simulink model "V2X_Core_SRI_coding_rate_symbol"  (R2023b)
settings: Solver=ode23tb  StartTime=0.0  StopTime=50  MaxStep=1e-2  RelTol=1e-3  AbsTol=1e-3
StopFcn:
  | run('saving.m')
values from neighbouring files (symbols this model uses):
  b = 1.6    [a2024_v2x_matlab_6veh.m]
  m = 2000    [a2024_v2x_matlab_6veh.m]
  mEgo = 1500    [a2024_v2x_matlab_6veh.m]
  Mode = 1    [a2024_v2x_matlab_6veh.m]    (also in v2x_matlab.m; v2x_matlabV2.m; v2x_matlab_6veh.m; v2x_matlab_R.m)
  RefSpeed = 90/3.6    (= 25)    [v2x_matlabV2.m]    (also in v2x_matlab_R.m)
  RelDistThreshold = 300    [v2x_matlabV2.m]    (also in v2x_matlab_R.m)
  s = RandStream("dsfmt19937","Seed",15)    [v2x_matlab.m]
  sampleTime = 0.1    [a2024_v2x_matlab_6veh.m]    (also in v2x_matlab.m; v2x_matlabV2.m; v2x_matlab_6veh.m; v2x_matlab_R.m)
  waypoints = [egoWP(:,2) egoWP(:,1), zeroforwp]    [a2024_v2x_matlab_6veh.m]    (also in misc.m = data.data.ActorSpecifications(1,1).Waypoints(:,[1,2]); v2x_matlab.m = data.data.ActorSpecifications(1,1).Waypoints(:,[1,2]); v2x_matlabV2.m = [5 -1.6 0; v2x_matlab_R.m = [5 -1.6 0)
  ZeroActors = struct(     'ActorID',0,     'Position', [1000 1000 1000],      'Velocity', [0 0 0],      'Roll', 0,      'Pitch', 0,      'Yaw', 0,      'AngularVelocity', [0 0 0])    [v2x_matlabV2.m]    (also in v2x_matlab_R.m)
undefined symbols (not defined in the file or in its folder): Battery, Brakes, Control, DiscIntNeverNeededParam, doppler, Drivetrain, ElectricMotor, Env, FB_flag, Init, SNR_value_list, Vehicle, Wheels
libraries: simulink x45, commofdm x29, commdigbbndam3 x15, commchan3 x14, simulink_extras x13, commcnvcod2 x12, commdigbbndpm3 x11, commblkintrlv2 x10, dspmathops x6, sharedtransform x6, autolibutils x6, autolibsharedcoupling x4
(part 8 of 8)

== matlab function V2X_Core_SRI_coding_rate_symbol/Calculate PDR/PDR V5/MATLAB Function ==
  settings: updateMethod=DISCRETE  sampleTime=sampleTime
  data: Tx input; PDR output; Rx input; Rx_out output; Msg_out output
function [PDR, Rx_out, Msg_out] = PDR(Tx, Rx)
    persistent N S prev_Rx
    if isempty(N) || isempty(S)
        N = 0;
        S = 0;
        prev_Rx = zeros(13,1);
    end
    if isequal(Tx, Rx) % Check if the entire vectors are the same
        N = N + 1;      % Increment the correct packet count
        prev_Rx = Rx;
        Rx_out = Rx;
        Msg_out = 1;
    else
        Rx_out = prev_Rx;
        Msg_out = 0;
    end
    S = S + 1;          % Increment the total count
    R = (N/S)*100;       % Calculate the packet delivery rate [%]
    PDR = [R; N; S];
end

== matlab function V2X_Core_SRI_coding_rate_symbol/Calculate PDR/PDR V5/MATLAB Function1 ==
  settings: sampleTime=sampleTime
  data: Vehicle_ID input; u input; y output double
function y = fcn(Vehicle_ID, u)

if isempty(u(:,Vehicle_ID)) 
    y = zeros(1,15);
else
    y = double(u(:,Vehicle_ID));
end

end

== matlab function V2X_Core_SRI_coding_rate_symbol/Calculate PDR/PDR V5/MATLAB Function2 ==
  settings: sampleTime=sampleTime
  data: Vehicle_ID input; u input; y output double
function y = fcn(Vehicle_ID, u)

if isempty(u(:,Vehicle_ID)) 
    y = zeros(1,15);
else
    y = double(u(:,Vehicle_ID));
end

end

== matlab function V2X_Core_SRI_coding_rate_symbol/VehicleDynamic/FiveSteteABS-TCS/Wheel Accel and Slip Estimator1/Kappa/MATLAB Function ==
  data: Omega input; xdot input; KappaEst output
function KappaEst = fcn(Omega, xdot)

Re = 0.29;
KappaEst = 0;
WhlSpd = Omega * Re;

if xdot*WhlSpd ~= 0
    KappaEst = (WhlSpd - xdot)/max([abs(xdot) abs(WhlSpd)]);
end

== matlab function V2X_Core_SRI_coding_rate_symbol/Calculate PDR/PDR V5/MATLAB Function6 ==
  data: u input; y output Bus: Actors; vehicleID input
function y = fcn(u,vehicleID)

actorsCount = size(u.Actors,1);

MinusOneActor = struct(...
    'ActorID',0,...
    'Position', [0 0 0], ...
    'Velocity', [0 0 0], ...
    'Roll', 0, ...
    'Pitch', 0, ...
    'Yaw', 0, ...
    'AngularVelocity', [0 0 0]);

if actorsCount < vehicleID
    y = MinusOneActor;
else
    y = u.Actors(vehicleID);
end
end

== matlab function V2X_Core_SRI_coding_rate_symbol/Calculate PDR/PDR V6/MATLAB Function ==
  settings: updateMethod=DISCRETE  sampleTime=sampleTime
  data: Tx input; PDR output; Rx input; Rx_out output; Msg_out output
function [PDR, Rx_out, Msg_out] = PDR(Tx, Rx)
    persistent N S prev_Rx
    if isempty(N) || isempty(S)
        N = 0;
        S = 0;
        prev_Rx = zeros(13,1);
    end
    if isequal(Tx, Rx) % Check if the entire vectors are the same
        N = N + 1;      % Increment the correct packet count
        prev_Rx = Rx;
        Rx_out = Rx;
        Msg_out = 1;
    else
        Rx_out = prev_Rx;
        Msg_out = 0;
    end
    S = S + 1;          % Increment the total count
    R = (N/S)*100;       % Calculate the packet delivery rate [%]
    PDR = [R; N; S];
end

== matlab function V2X_Core_SRI_coding_rate_symbol/Calculate PDR/PDR V6/MATLAB Function1 ==
  settings: sampleTime=sampleTime
  data: Vehicle_ID input; u input; y output double
function y = fcn(Vehicle_ID, u)

if isempty(u(:,Vehicle_ID)) 
    y = zeros(1,15);
else
    y = double(u(:,Vehicle_ID));
end

end

== matlab function V2X_Core_SRI_coding_rate_symbol/Calculate PDR/PDR V6/MATLAB Function2 ==
  settings: sampleTime=sampleTime
  data: Vehicle_ID input; u input; y output double
function y = fcn(Vehicle_ID, u)

if isempty(u(:,Vehicle_ID)) 
    y = zeros(1,15);
else
    y = double(u(:,Vehicle_ID));
end

end

== matlab function V2X_Core_SRI_coding_rate_symbol/Calculate PDR/PDR V6/MATLAB Function6 ==
  data: u input; y output Bus: Actors; vehicleID input
function y = fcn(u,vehicleID)

actorsCount = size(u.Actors,1);

MinusOneActor = struct(...
    'ActorID',0,...
    'Position', [0 0 0], ...
    'Velocity', [0 0 0], ...
    'Roll', 0, ...
    'Pitch', 0, ...
    'Yaw', 0, ...
    'AngularVelocity', [0 0 0]);

if actorsCount < vehicleID
    y = MinusOneActor;
else
    y = u.Actors(vehicleID);
end
end

== matlab function V2X_Core_SRI_coding_rate_symbol/DSRC/Subsystem/MATLAB Function3 ==
  settings: sampleTime=sampleTime
  data: input input; Actors output
function Actors = getRealValues(input) 

modulated = input;

NumActors = modulated(1,:);
Time = modulated(2,:);

ActorID = modulated(3,1);

posMultip = 10;  % 10
posX = (modulated(4,:)/posMultip);
posY = (modulated(5,:)/posMultip);
posZ = (modulated(6,:)/posMultip);

velMultip = 50;  % 50
vX = (modulated(7,:)/velMultip);
vY = (modulated(8,:)/velMultip);
vZ = (modulated(9,:)/velMultip);

rpyMultip = 50;  % 50
Roll = (modulated(10,:)/rpyMultip);
Pitch = (modulated(11,:)/rpyMultip);
Yaw = (modulated(12,:)/rpyMultip);

angvelMultip = 50;  % 50
angularVelocityX = (modulated(13,:)/angvelMultip);
angularVelocityY = (modulated(14,:)/angvelMultip);
angularVelocityZ = (modulated(15,:)/angvelMultip);

% Velocity = [vX vY vZ];
% Position = [posX posY posZ];
% AngularVelocity = [angularVelocityX; angularVelocityY; angularVelocityZ];


%Actors = [NumActors; Time; ActorID; Position; Velocity; Roll; Pitch; Yaw; AngularVelocity];
Actors = double([NumActors; Time; ActorID; posX; posY; posZ; vX; vY; vZ; Roll; Pitch; Yaw; angularVelocityX; angularVelocityY; angularVelocityZ]);


end

== matlab function V2X_Core_SRI_coding_rate_symbol/DSRC/Subsystem4/MATLAB Function3 ==
  settings: sampleTime=sampleTime
  data: input input; Actors output
function Actors = getRealValues(input) 

modulated = input;

NumActors = modulated(1,:);
Time = modulated(2,:);

ActorID = modulated(3,1);

posMultip = 10;  % 10
posX = (modulated(4,:)/posMultip);
posY = (modulated(5,:)/posMultip);
posZ = (modulated(6,:)/posMultip);

velMultip = 50;  % 50
vX = (modulated(7,:)/velMultip);
vY = (modulated(8,:)/velMultip);
vZ = (modulated(9,:)/velMultip);

rpyMultip = 50;  % 50
Roll = (modulated(10,:)/rpyMultip);
Pitch = (modulated(11,:)/rpyMultip);
Yaw = (modulated(12,:)/rpyMultip);

angvelMultip = 50;  % 50
angularVelocityX = (modulated(13,:)/angvelMultip);
angularVelocityY = (modulated(14,:)/angvelMultip);
angularVelocityZ = (modulated(15,:)/angvelMultip);

% Velocity = [vX vY vZ];
% Position = [posX posY posZ];
% AngularVelocity = [angularVelocityX; angularVelocityY; angularVelocityZ];


%Actors = [NumActors; Time; ActorID; Position; Velocity; Roll; Pitch; Yaw; AngularVelocity];
Actors = double([NumActors; Time; ActorID; posX; posY; posZ; vX; vY; vZ; Roll; Pitch; Yaw; angularVelocityX; angularVelocityY; angularVelocityZ]);


end

== matlab function V2X_Core_SRI_coding_rate_symbol/DSRC/Subsystem7/MATLAB Function1 ==
  settings: sampleTime=inherited
  data: busActors3Test1 input; Actor output int16 size=15; VehicleID input; VehicleData output Bus: Actors; EgoData input Bus: Actors; counter_out output; SNR output; Pr output
  events: trigger input RISING_EDGE_EVENT
function [Actor, VehicleData, counter_out, SNR, Pr]  = convBus2IntVector(busActors3Test1, VehicleID, EgoData)

% Data extracted from actorss bus

%ActorId = BusActors1Actors.Actors(ActorID).ActorID(1:1);
numActors = busActors3Test1.NumActors;
%time = busActors3Test1.Time;
time = busActors3Test1.Time;

ActorID = VehicleID;

posX = busActors3Test1.Actors(ActorID).Position(1:1);
posY = busActors3Test1.Actors(ActorID).Position(2:2);
posZ = busActors3Test1.Actors(ActorID).Position(3:3);
vPos = [posX posY posZ];

vX = busActors3Test1.Actors(ActorID).Velocity(1:1);
vY = busActors3Test1.Actors(ActorID).Velocity(2:2);
vZ = busActors3Test1.Actors(ActorID).Velocity(3:3);

roll = busActors3Test1.Actors(ActorID).Roll(1:1);
pitch = busActors3Test1.Actors(ActorID).Pitch(1:1);
yaw = busActors3Test1.Actors(ActorID).Yaw(1:1);


angularVelocityX = busActors3Test1.Actors(ActorID).AngularVelocity(1:1);
angularVelocityY = busActors3Test1.Actors(ActorID).AngularVelocity(2:2);
angularVelocityZ = busActors3Test1.Actors(ActorID).AngularVelocity(3:3);

VehicleData = busActors3Test1.Actors(VehicleID);


%% Converting the data

ActorID = int16(ActorID);

posMultip = 10;
posX = int16(round(posMultip*posX));
posY = int16(round(posMultip*posY));
posZ = int16(round(posMultip*posZ));

velMultip = 50;
vX = int16(round(velMultip * vX));
vY = int16(round(velMultip * vY));
vZ = int16(round(velMultip * vZ));

rpyMultip = 50;
roll = int16(round(rpyMultip * roll));
pitch = int16(round(rpyMultip * pitch));
yaw = int16(round(rpyMultip * yaw));

angvelMultip = 50;
angularVelocityX = int16(round(angvelMultip * angularVelocityX));
angularVelocityY = int16(round(angvelMultip * angularVelocityY));
angularVelocityZ = int16(round(angvelMultip * angularVelocityZ));


% Output vector
%zerosVector = zeros(9,1);

intVector = [numActors; time; ActorID; posX; posY; posZ; vX; vY; vZ; roll; pitch; yaw; angularVelocityX; angularVelocityY; angularVelocityZ];


%% Pathloss (freespace)

EgoPos = EgoData.Position;
dist = norm(vPos - EgoPos);

fc = 5.9e9;  % Carrier frequency
lambda = (physconst('LightSpeed'))/fc;

PL = fspl(dist, lambda);

Pt_dBm = 33;    % [dBm] Transmission power; maximum permissible transmit power level
Pt_dbW = Pt_dBm - 30;
sigma = rand(1) + 3.2;  % [3.7 +- 0.5] Variance of the shadowing effect in the wireless communication channel
                        % shadowing follows a log-normal random distribution
X = 2*rand(1)-1;      % random variable following a normal distribution with mean 0 and standard deviation 1
SH = sigma * X;

% h_T = 1;
% h_R = 1;
% dF =  (4*h_T*h_R)/lambda
% lambda1 = 1.61; % Pathloss exponent LOS
% lambda2 = 1.85; % Pathloss exponent NLOS

Pr = Pt_dBm - PL - SH; 

% l1 = 10*lambda1*log(dF)
% l2 = 10*lambda2*log(dist/dF)
% Pr = Prt - l1 - l2 + SH;

P_SEN = -60;

%ZeroActors = int16(zeros(15,1));
% 
% counter = 0;
% storedPacket = int16(nan(15,1));
% 
% if Pr > P_SEN
%     Actor = intVector;
%     storedPacket = intVector;
%     counter = 0;
% elseif counter < 10
%     Actor = storedPacket;
%     counter = counter + 1;
% end


%disp(storedPacket)


% persistent prev_value;
% if isempty(prev_value)
%     prev_value = int16(nan(15,1)); % Initialize to a default value
% end
% 
% if Pr > P_SEN
%     Actor = intVector;
%     prev_value = intVector;
%     counter = 0;
% elseif counter < 1
%     Actor = prev_value;
%     counter = counter + 1;
% end

Actor = intVector;
%% SNR
bandwidth = 10e6;
F = 6; % [dB] Noise figure
k = physconst('Boltzmann'); % Boltzmann állandó
T = 300; % [K] Abszolút hőmérséklet

N0 = bandwidth *k*T;
N0dbm = 10 * log10(1000*N0);
N0dbW = N0dbm - 30; 
%N0 = -99;
SNR = Pr - N0dbm;
%signalpower = Pr;s


%% Packet counter
persistent counter
if isempty(counter)
    counter = 0;
end

if (Pr > P_SEN)
    counter = counter + 1;
end

counter_out = counter;
end

== matlab function V2X_Core_SRI_coding_rate_symbol/DSRC/Subsystem7/MATLAB Function2 ==
  settings: updateMethod=DISCRETE  sampleTime=sampleTime
  data: modulated input; signal output; SNR input
function signal = PRO_error(modulated, SNR)

signal = awgn(modulated,SNR);

== matlab function V2X_Core_SRI_coding_rate_symbol/DSRC/Subsystem7/MATLAB Function3 ==
  settings: sampleTime=sampleTime
  data: input input; Actors output
function Actors = getRealValues(input) 

modulated = input;

NumActors = modulated(1,:);
Time = modulated(2,:);

ActorID = modulated(3,1);

posMultip = 10;  % 10
posX = (modulated(4,:)/posMultip);
posY = (modulated(5,:)/posMultip);
posZ = (modulated(6,:)/posMultip);

velMultip = 50;  % 50
vX = (modulated(7,:)/velMultip);
vY = (modulated(8,:)/velMultip);
vZ = (modulated(9,:)/velMultip);

rpyMultip = 50;  % 50
Roll = (modulated(10,:)/rpyMultip);
Pitch = (modulated(11,:)/rpyMultip);
Yaw = (modulated(12,:)/rpyMultip);

angvelMultip = 50;  % 50
angularVelocityX = (modulated(13,:)/angvelMultip);
angularVelocityY = (modulated(14,:)/angvelMultip);
angularVelocityZ = (modulated(15,:)/angvelMultip);

% Velocity = [vX vY vZ];
% Position = [posX posY posZ];
% AngularVelocity = [angularVelocityX; angularVelocityY; angularVelocityZ];


%Actors = [NumActors; Time; ActorID; Position; Velocity; Roll; Pitch; Yaw; AngularVelocity];
Actors = double([NumActors; Time; ActorID; posX; posY; posZ; vX; vY; vZ; Roll; Pitch; Yaw; angularVelocityX; angularVelocityY; angularVelocityZ]);


end

== matlab function V2X_Core_SRI_coding_rate_symbol/DSRC/Subsystem8/MATLAB Function3 ==
  settings: sampleTime=sampleTime
  data: input input; Actors output
function Actors = getRealValues(input) 

modulated = input;

NumActors = modulated(1,:);
Time = modulated(2,:);

ActorID = modulated(3,1);

posMultip = 10;  % 10
posX = (modulated(4,:)/posMultip);
posY = (modulated(5,:)/posMultip);
posZ = (modulated(6,:)/posMultip);

velMultip = 50;  % 50
vX = (modulated(7,:)/velMultip);
vY = (modulated(8,:)/velMultip);
vZ = (modulated(9,:)/velMultip);

rpyMultip = 50;  % 50
Roll = (modulated(10,:)/rpyMultip);
Pitch = (modulated(11,:)/rpyMultip);
Yaw = (modulated(12,:)/rpyMultip);

angvelMultip = 50;  % 50
angularVelocityX = (modulated(13,:)/angvelMultip);
angularVelocityY = (modulated(14,:)/angvelMultip);
angularVelocityZ = (modulated(15,:)/angvelMultip);

% Velocity = [vX vY vZ];
% Position = [posX posY posZ];
% AngularVelocity = [angularVelocityX; angularVelocityY; angularVelocityZ];


%Actors = [NumActors; Time; ActorID; Position; Velocity; Roll; Pitch; Yaw; AngularVelocity];
Actors = double([NumActors; Time; ActorID; posX; posY; posZ; vX; vY; vZ; Roll; Pitch; Yaw; angularVelocityX; angularVelocityY; angularVelocityZ]);


end

== matlab function V2X_Core_SRI_coding_rate_symbol/DSRC/Subsystem3/2//3 64 QAM/MATLAB Function3 ==
  settings: updateMethod=DISCRETE
  data: input input; output output
function output = removeZeros(input)

output = input(1:40,:,:);

end

== matlab function V2X_Core_SRI_coding_rate_symbol/MATLAB Function ==
  settings: updateMethod=DISCRETE
  data: Rel_Dist input; TTC output; Rel_Vel input; FB_Flag output
function [TTC, FB_Flag] = TTC_Flag(Rel_Dist, Rel_Vel)

persistent fflag  ffb_flag 

if isempty(fflag)
    fflag = 1;
    ffb_flag = 0;
    TTC = 10;
else
    TTC = Rel_Dist / Rel_Vel;
    if TTC < 1.5
        ffb_flag = 1;
    end
end
FB_Flag = ffb_flag;

end

== matlab function V2X_Core_SRI_coding_rate_symbol/MATLAB Function8 ==
  settings: updateMethod=DISCRETE  sampleTime=sampleTime
  data: u input; RelDist output
function RelDist = fcn(u)

for i = 1:10
    RelDist = 100;
end

RelDist = u;

== matlab function V2X_Core_SRI_coding_rate_symbol/DSRC/Subsystem3/2//3 64 QAM1/MATLAB Function3 ==
  settings: updateMethod=DISCRETE
  data: input input; output output
function output = removeZeros(input)

output = input(1:40,:,:);

end

== matlab function V2X_Core_SRI_coding_rate_symbol/MATLAB Function1 ==
  settings: updateMethod=DISCRETE  sampleTime=sampleTime
  data: u input; RelDist output
function RelDist = fcn(u)

persistent counter

if isempty(counter)
    counter = 0;
end

if counter < 20
    counter = counter + 1;
    RelDist = 10;
else
    RelDist = u;
end

== matlab function V2X_Core_SRI_coding_rate_symbol/Vehicle 2/MATLAB Function1 ==
  data: busActors3Test1 input; intVector output int16 size=15; VehicleID input
  events: trigger input RISING_EDGE_EVENT
function intVector = convBus2IntVector(busActors3Test1, VehicleID)

% Data extracted from actorss bus

%ActorId = BusActors1Actors.Actors(ActorID).ActorID(1:1);
numActors = busActors3Test1.NumActors;
time = busActors3Test1.Time;

ActorID = VehicleID;

posX = busActors3Test1.Actors(ActorID).Position(1:1);
posY = busActors3Test1.Actors(ActorID).Position(2:2);
posZ = busActors3Test1.Actors(ActorID).Position(3:3);

vX = busActors3Test1.Actors(ActorID).Velocity(1:1);
vY = busActors3Test1.Actors(ActorID).Velocity(2:2);
vZ = busActors3Test1.Actors(ActorID).Velocity(3:3);

roll = busActors3Test1.Actors(ActorID).Roll(1:1);
pitch = busActors3Test1.Actors(ActorID).Pitch(1:1);
yaw = busActors3Test1.Actors(ActorID).Yaw(1:1);


angularVelocityX = busActors3Test1.Actors(ActorID).AngularVelocity(1:1);
angularVelocityY = busActors3Test1.Actors(ActorID).AngularVelocity(2:2);
angularVelocityZ = busActors3Test1.Actors(ActorID).AngularVelocity(3:3);


% Converting the data

ActorID = int16(ActorID);

posMultip = 10;
posX = int16(round(posMultip*posX));
posY = int16(round(posMultip*posY));
posZ = int16(round(posMultip*posZ));

velMultip = 50;
vX = int16(round(velMultip * vX));
vY = int16(round(velMultip * vY));
vZ = int16(round(velMultip * vZ));

rpyMultip = 50;
roll = int16(round(rpyMultip * roll));
pitch = int16(round(rpyMultip * pitch));
yaw = int16(round(rpyMultip * yaw));

angvelMultip = 50;
angularVelocityX = int16(round(angvelMultip * angularVelocityX));
angularVelocityY = int16(round(angvelMultip * angularVelocityY));
angularVelocityZ = int16(round(angvelMultip * angularVelocityZ));


% Output vector
%zerosVector = zeros(9,1);

intVector = [numActors; time; ActorID; posX; posY; posZ; vX; vY; vZ; roll; pitch; yaw; angularVelocityX; angularVelocityY; angularVelocityZ];
end

== matlab function V2X_Core_SRI_coding_rate_symbol/DSRC/Subsystem/MATLAB Function1 ==
  settings: sampleTime=inherited
  data: busActors3Test1 input; Actor output int16 size=15; VehicleID input; VehicleData output Bus: Actors; EgoData input Bus: Actors; counter_out output; SNR output; Pr output; data input
  events: trigger input RISING_EDGE_EVENT
function [Actor, VehicleData, counter_out, SNR, Pr]  = convBus2IntVector(busActors3Test1, VehicleID, EgoData, data)

% Data extracted from actorss bus

%ActorId = BusActors1Actors.Actors(ActorID).ActorID(1:1);
numActors = busActors3Test1.NumActors;
%time = busActors3Test1.Time;
time = busActors3Test1.Time;

ActorID = VehicleID;

posX = busActors3Test1.Actors(ActorID).Position(1:1);
posY = busActors3Test1.Actors(ActorID).Position(2:2);
posZ = busActors3Test1.Actors(ActorID).Position(3:3);
vPos = [posX posY posZ];

vX = busActors3Test1.Actors(ActorID).Velocity(1:1);
vY = busActors3Test1.Actors(ActorID).Velocity(2:2);
vZ = busActors3Test1.Actors(ActorID).Velocity(3:3);

roll = busActors3Test1.Actors(ActorID).Roll(1:1);
pitch = busActors3Test1.Actors(ActorID).Pitch(1:1);
yaw = busActors3Test1.Actors(ActorID).Yaw(1:1);


angularVelocityX = busActors3Test1.Actors(ActorID).AngularVelocity(1:1);
angularVelocityY = busActors3Test1.Actors(ActorID).AngularVelocity(2:2);
angularVelocityZ = busActors3Test1.Actors(ActorID).AngularVelocity(3:3);

VehicleData = busActors3Test1.Actors(VehicleID);


%% Converting the data

ActorID = int16(ActorID);

posMultip = 10;
posX = int16(round(posMultip*posX));
posY = int16(round(posMultip*posY));
posZ = int16(round(posMultip*posZ));

velMultip = 50;
vX = int16(round(velMultip * vX));
vY = int16(round(velMultip * vY));
vZ = int16(round(velMultip * vZ));

rpyMultip = 50;
roll = int16(round(rpyMultip * roll));
pitch = int16(round(rpyMultip * pitch));
yaw = int16(round(rpyMultip * yaw));

angvelMultip = 50;
angularVelocityX = int16(round(angvelMultip * angularVelocityX));
angularVelocityY = int16(round(angvelMultip * angularVelocityY));
angularVelocityZ = int16(round(angvelMultip * angularVelocityZ));


% Output vector
%zerosVector = zeros(9,1);

intVector = [numActors; time; ActorID; posX; posY; posZ; vX; vY; vZ; roll; pitch; yaw; angularVelocityX; angularVelocityY; angularVelocityZ];


%% Pathloss (freespace)

EgoPos = EgoData.Position;
dist = norm(vPos - EgoPos);

fc = 5.9e9;  % Carrier frequency
lambda = (physconst('LightSpeed'))/fc;

PL = fspl(dist, lambda);

Pt_dBm = 23;    % [dBm] Transmission power; maximum permissible transmit power level
Pt_dbW = Pt_dBm - 30;
sigma = rand(1) + 3.2;  % [3.7 +- 0.5] Variance of the shadowing effect in the wireless communication channel
                        % shadowing follows a log-normal random distribution
X = 2*rand(1)-1;      % random variable following a normal distribution with mean 0 and standard deviation 1
SH = sigma * X;

% h_T = 1;
% h_R = 1;
% dF =  (4*h_T*h_R)/lambda
% lambda1 = 1.61; % Pathloss exponent LOS
% lambda2 = 1.85; % Pathloss exponent NLOS

Pr = Pt_dBm - PL - SH; 

% l1 = 10*lambda1*log(dF)
% l2 = 10*lambda2*log(dist/dF)
% Pr = Prt - l1 - l2 + SH;
if data == 1
    P_SEN = -60;
else
    P_SEN = -80;
end
%P_SEN = -60;

%ZeroActors = int16(zeros(15,1));
% 
% counter = 0;
% storedPacket = int16(nan(15,1));
% 
% if Pr > P_SEN
%     Actor = intVector;
%     storedPacket = intVector;
%     counter = 0;
% elseif counter < 10
%     Actor = storedPacket;
%     counter = counter + 1;
% end


%disp(storedPacket)


% persistent prev_value;
% if isempty(prev_value)
%     prev_value = int16(nan(15,1)); % Initialize to a default value
% end
% 
% if Pr > P_SEN
%     Actor = intVector;
%     prev_value = intVector;
%     counter = 0;
% elseif counter < 1
%     Actor = prev_value;
%     counter = counter + 1;
% end

Actor = intVector;
%% SNR
bandwidth = 10e6;
F = 6; % [dB] Noise figure
k = physconst('Boltzmann'); % Boltzmann állandó
T = 300; % [K] Abszolút hőmérséklet

N0 = bandwidth *k*T;
N0dbm = 10 * log10(1000*N0);
N0dbW = N0dbm - 30; 
%N0 = -99;
SNR = Pr - N0dbm;
%signalpower = Pr;s


%% Packet counter
persistent counter
if isempty(counter)
    counter = 0;
end

if (Pr > P_SEN)
    counter = counter + 1;
end

counter_out = counter;
end
